simulink model "MOT_CTRL_PTH_FUN_001_2"  (R2025a)
settings: Solver=VariableStepAuto  StartTime=0.0  StopTime=10.0  RelTol=1e-3
settings Model: DataDictionary=Hbridge.sldd  Creator=tecnicomcbti  LastModifiedBy=tecnicomcbti

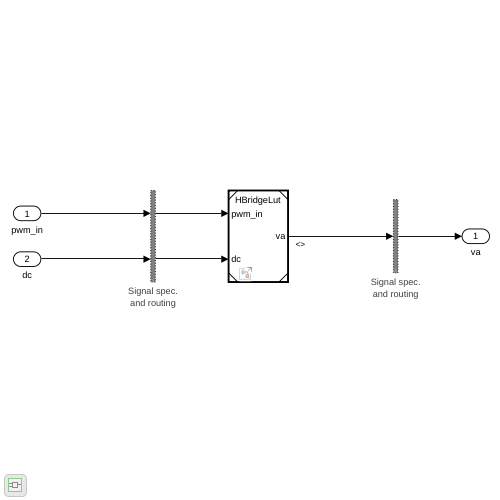
[thumbnail: Simulink's stored preview of the top-level diagram]
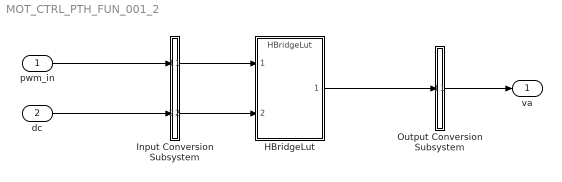
== system MOT_CTRL_PTH_FUN_001_2 ==
  pwm_in : Inport  OutDataTypeStr=double  PortDimensions=[1]  SampleTime=0
  dc : Inport  Port=2  OutDataTypeStr=double  PortDimensions=[1]  SampleTime=0
  HBridgeLut : ModelReference  ModelNameDialog=HBridgeLut  SimulationMode=Normal  ModelReferenceVersion=1.7
  Input Conversion Subsystem : Subsystem  Tag=__SLT_ICS__  Description=|
      | Signal spec.
      | and routing
      settings: AttributesFormatString=%<Description>
  Output Conversion Subsystem : Subsystem  Tag=__SLT_OCS__  Description=|
      | Signal spec.
      | and routing
      settings: AttributesFormatString=%<Description>
  va : Outport
  wires:
  pwm_in/1 -> Input Conversion Subsystem/1(Inport_1)
  dc/1 -> Input Conversion Subsystem/2(Inport_2)
  Output Conversion Subsystem/1(Outport_1) -> va/1
  Input Conversion Subsystem/1(Outport_1) -> HBridgeLut/1
  Input Conversion Subsystem/2(Outport_2) -> HBridgeLut/2
  HBridgeLut/1 -> Output Conversion Subsystem/1(Inport_1)

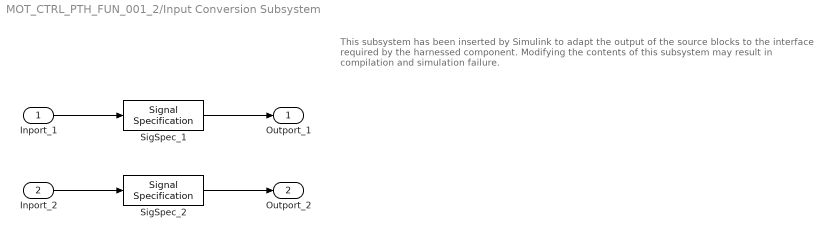
== system MOT_CTRL_PTH_FUN_001_2/Input Conversion Subsystem ==
  note: This subsystem has been inserted by Simulink to adapt the output of the source blocks to the interface required by the harnessed component.
      |  Modifying the contents of this subsystem may result in compilation and simulation failure.
  Inport_1 : Inport
  Inport_2 : Inport  Port=2
  SigSpec_1 : SignalSpecification  OutDataTypeStr=double  Dimensions=[1]  SampleTime=[0, 0]
  SigSpec_2 : SignalSpecification  OutDataTypeStr=double  Dimensions=[1]  SampleTime=[0, 0]
  Outport_1 : Outport
  Outport_2 : Outport  Port=2
  wires:
  SigSpec_1/1 -> Outport_1/1
  Inport_1/1 -> SigSpec_1/1
  SigSpec_2/1 -> Outport_2/1
  Inport_2/1 -> SigSpec_2/1

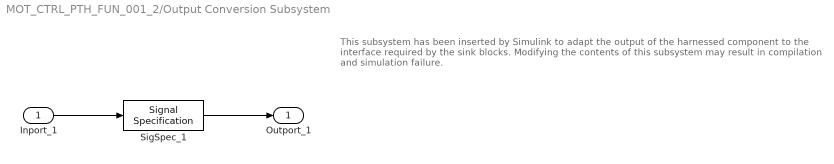
== system MOT_CTRL_PTH_FUN_001_2/Output Conversion Subsystem ==
  note: This subsystem has been inserted by Simulink to adapt the output of the harnessed component to the interface required by the sink blocks.
      |  Modifying the contents of this subsystem may result in compilation and simulation failure.
  Inport_1 : Inport
  SigSpec_1 : SignalSpecification  OutDataTypeStr=double  Dimensions=[1]
  Outport_1 : Outport
  wires:
  Inport_1/1 -> SigSpec_1/1
  SigSpec_1/1 -> Outport_1/1
